simulink model "generate_elbow_motion"  (R2025a)
settings: Solver=FixedStepDiscrete  StartTime=0.0  StopTime=inf  FixedStep=0.01  RelTol=1e-3
PreLoadFcn:
  | frs = FrankaRobotSettings();
libraries: franka_simulink x1
settings Model: SimulationMode=external  ExtModeTrigDuration=10000  Creator=vasi_ko  LastModifiedBy=kvasios
settings SolverCC: ConcurrentTasks=on  AlgebraicLoopSolver=TrustRegion  AutoInsertRateTranBlk=on
settings DataIOCC: LimitDataPoints=on  SaveFormat=Array  ReturnWorkspaceOutputs=off
settings OptimizationCC: EnhancedBackFolding=on  PassReuseOutputArgsAs=Individual arguments  ZeroExternalMemoryAtStartup=off  ZeroInternalMemoryAtStartup=off  MaxStackSize=200000  OptimizeBlockOrder=speed  DifferentSizesBufferReuse=on  OptimizationCustomize=off  EfficientTunableParamExpr=on
settings DebuggingCC: SolverPrmCheckMsg=warning  ParameterTunabilityLossMsg=error  UnconnectedInputMsg=warning  UnconnectedOutputMsg=warning  UnconnectedLineMsg=warning  SFUnexpectedBacktrackingDiag=warning  SFNoUnconditionalDefaultTransitionDiag=warning  SFExecutionAtInitializationDiag=none  ArithmeticOperatorsInVariantConditions=warning
settings HardwareCC: ProdBitPerLong=64.0  ProdLargestAtomicInteger=LongLong  ProdLargestAtomicFloat=Double  ProdLongLongMode=on  ProdHWDeviceType=ARM Compatible->ARM Cortex-A (64-bit)
settings ModelReferenceCC: EnableRefExpFcnMdlSchedulingChecks=on  PropagateSignalLabelsOutOfModel=off
settings SFSimCC: SimUseLocalCustomCode=off  MATLABDynamicMemAlloc=off  CustomCodeUndefinedFunction=UseInterfaceOnly  SimTargetLang=C++  SimDLTargetLibrary=mkl-dnn
settings RTWCC: SystemTargetFile=ert.tlc  HardwareBoard=NVIDIA Jetson  TLCOptions="-aInlineSetEventsForThisBaseRateFcn=TLC_FALSE -aSuppressMultiTaskScheduler=TLC_FALSE  -aRateBasedStepFcn=0"  TemplateMakefile=ert_default_tmf  RTWVerbose=off  RTWUseLocalCustomCode=off  BuildConfiguration=Faster Runs  TargetLang=C++  GPUComputeCapability=3.5  DLArmComputeVersion=19.05  Description=Embedded Coder
settings CodeAppCC: ForceParamTrailComments=on  IgnoreCustomStorageClasses=off  OperatorAnnotations=on  SimulinkDataObjDesc=on  SFDataObjDesc=on  InsertBlockDesc=on
settings ERTTargetCC: ExtModeTransport=0.0  ExtModeMexFile=ext_comm  ExtModeIntrfLevel=Level1  InlinedParameterPlacement=Hierarchical  RootIOFormat=Structure reference  TargetLangStandard=C++14 (ISO)
settings ConfigComp: CovMetricSettings=dw  CovSaveCumulativeToWorkspaceVar=on  CovSaveSingleToWorkspaceVar=on  CovExternalEMLEnable=off  CovSFcnEnable=off

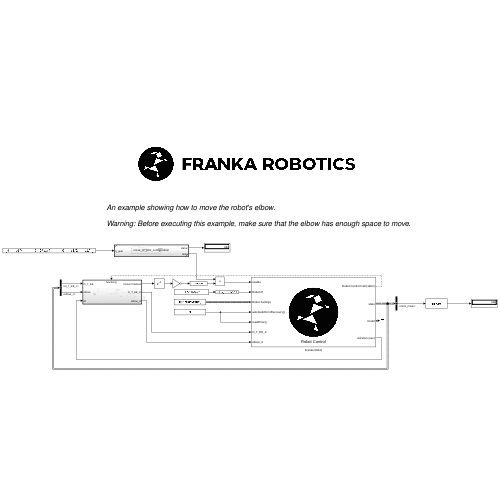
[thumbnail: Simulink's stored preview of the top-level diagram]
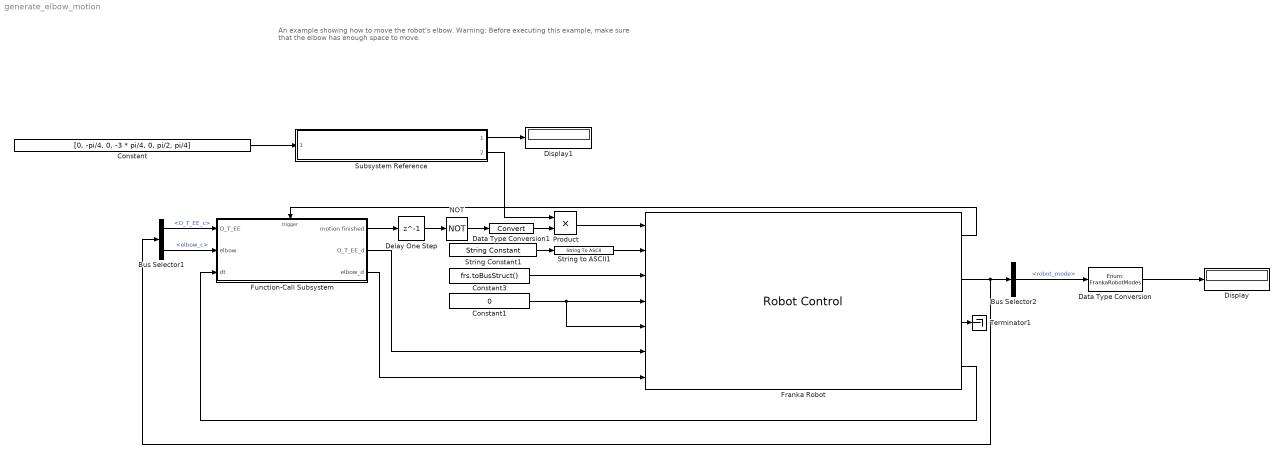
== system generate_elbow_motion ==
  note: An example showing how to move the robot's elbow.
      |
      | Warning: Before executing this example, make sure that the elbow has enough space to move.
  Bus Selector1 : BusSelector  OutputSignals=O_T_EE_c,elbow_c
  Bus Selector2 : BusSelector  OutputSignals=robot_mode
  Constant : Constant  Value=[0, -pi/4, 0, -3 * pi/4, 0, pi/2, pi/4]
  Constant1 : Constant  Value=0  OutDataTypeStr=Inherit: Inherit via back propagation
  Constant3 : Constant  Value=frs.toBusStruct()  OutDataTypeStr=Bus: FrankaRobotSettingsBus
  Data Type Conversion : DataTypeConversion  OutDataTypeStr=Enum: FrankaRobotModes  SaturateOnIntegerOverflow=off  RndMeth=Floor
  Data Type Conversion1 : DataTypeConversion  SaturateOnIntegerOverflow=off  RndMeth=Floor
  Delay One Step : Delay  DelayLength=1
  Display : Display
  Display1 : Display
  Franka Robot : franka_simulink/Robot Control  control_mode=Cartesian Pose
      settings: SourceProductName=Franka Robotics Simulink Support Package
  Function-Call Subsystem : Subsystem  TreatAsAtomicUnit=on
      settings: RTWSystemCode=Nonreusable function
  NOT : Logic  Operator=NOT  IconShape=distinctive  AllPortsSameDT=off  OutDataTypeStr=boolean
  Product : Product
  String Constant1 : StringConstant  String="\"172.16.0.2\""
  String to ASCII1 : StringToASCII  OutputVectorSize=16
  Subsystem Reference : Subsystem  TreatAsAtomicUnit=on  ReferencedSubsystem=move_to_joint_configuration
  Terminator1 : Terminator
  wires:
  Constant/1 -> Subsystem Reference/1
  Bus Selector2/1 -> Data Type Conversion/1  "<robot_mode>"
  Constant3/1 -> Franka Robot/3
  Franka Robot/4 -> Function-Call Subsystem/3(dt)
  Product/1 -> Franka Robot/1
  Function-Call Subsystem/1(motion finished) -> Delay One Step/1
  Constant1/1 -> Franka Robot/5, Franka Robot/4
  NOT/1 -> Data Type Conversion1/1
  Data Type Conversion1/1 -> Product/2
  Franka Robot/3 -> Terminator1/1
  Bus Selector1/1 -> Function-Call Subsystem/1(O_T_EE)  "<O_T_EE_c>"
  Function-Call Subsystem/2(O_T_EE_d) -> Franka Robot/6
  Subsystem Reference/2 -> Product/1
  Franka Robot/1 -> Function-Call Subsystem/Trigger
  Delay One Step/1 -> NOT/1
  Data Type Conversion/1 -> Display/1
  Franka Robot/2 -> Bus Selector1/1, Bus Selector2/1
  String Constant1/1 -> String to ASCII1/1
  Subsystem Reference/1 -> Display1/1
  String to ASCII1/1 -> Franka Robot/2
  Function-Call Subsystem/3(elbow_d) -> Franka Robot/7
  Bus Selector1/2 -> Function-Call Subsystem/2(elbow)  "<elbow_c>"

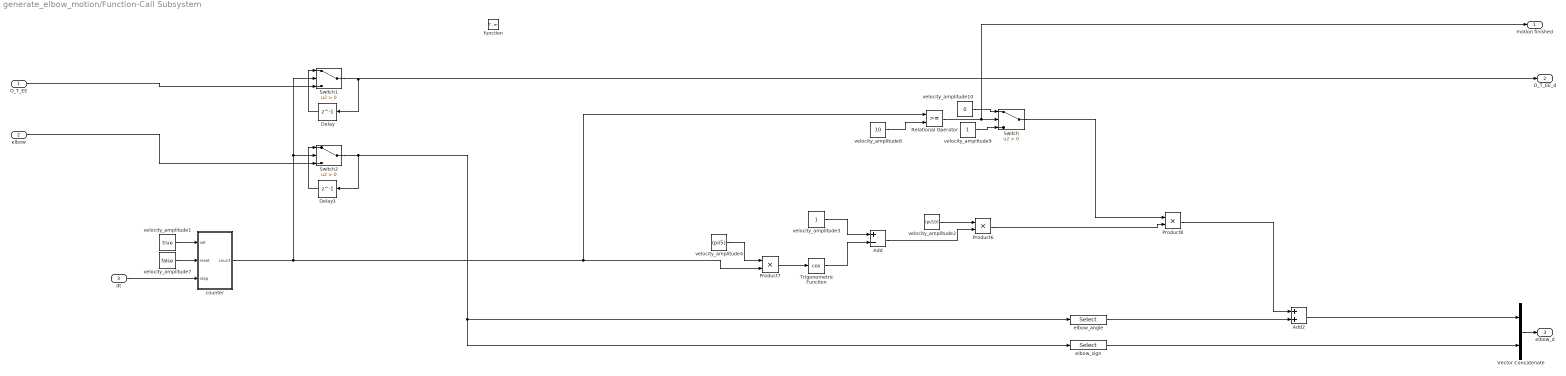
== system generate_elbow_motion/Function-Call Subsystem ==
  O_T_EE : Inport
  elbow : Inport  Port=2
  dt : Inport  Port=3
  function : TriggerPort  TriggerType=function-call  VariantControl=(inherit)
  Add : Sum  Inputs=+-
  Add2 : Sum
  Delay : Delay  DelayLength=1
  Delay1 : Delay  DelayLength=1
  Product6 : Product
  Product7 : Product
  Product8 : Product
  Relational Operator : RelationalOperator  OutDataTypeStr=boolean  InputSameDT=off
  Switch : Switch  Criteria=u2 > Threshold  SaturateOnIntegerOverflow=off  InputSameDT=off
  Switch1 : Switch  Criteria=u2 > Threshold  SaturateOnIntegerOverflow=off  InputSameDT=off
  Switch2 : Switch  Criteria=u2 > Threshold  SaturateOnIntegerOverflow=off  InputSameDT=off
  Trigonometric Function : Trigonometry  Operator=cos  NumberOfIterations=50
  Vector Concatenate : Concatenate
  counter : Subsystem
  elbow_angle : Selector  InputPortWidth=2  IndexOptions=Index vector (dialog)  Indices=1  OutputSizes=1
  elbow_sign : Selector  InputPortWidth=2  IndexOptions=Index vector (dialog)  Indices=2  OutputSizes=1
  velocity_amplitude1 : Constant  Value=true  VectorParams1D=off
  velocity_amplitude10 : Constant  Value=0  VectorParams1D=off
  velocity_amplitude2 : Constant  Value=(pi/10)  VectorParams1D=off
  velocity_amplitude3 : Constant  VectorParams1D=off
  velocity_amplitude4 : Constant  Value=(pi/5)  VectorParams1D=off
  velocity_amplitude7 : Constant  Value=false  VectorParams1D=off
  velocity_amplitude8 : Constant  Value=10  VectorParams1D=off
  velocity_amplitude9 : Constant  VectorParams1D=off
  motion finished : Outport  VectorParamsAs1DForOutWhenUnconnected=off
  O_T_EE_d : Outport  Port=2  VectorParamsAs1DForOutWhenUnconnected=off
  elbow_d : Outport  Port=3  VectorParamsAs1DForOutWhenUnconnected=off
  wires:
  elbow_angle/1 -> Add2/2
  elbow/1 -> Switch2/3
  Add/1 -> Product6/2
  velocity_amplitude7/1 -> counter/2(reset)
  counter/1(count) -> Relational Operator/1, Product7/2, Switch1/2, Switch2/2
  elbow_sign/1 -> Vector Concatenate/2
  Delay/1 -> Switch1/1
  Switch2/1 -> elbow_angle/1, elbow_sign/1, Delay1/1
  velocity_amplitude8/1 -> Relational Operator/2
  Switch1/1 -> O_T_EE_d/1, Delay/1
  velocity_amplitude4/1 -> Product7/1
  Product8/1 -> Add2/1
  velocity_amplitude9/1 -> Switch/3
  O_T_EE/1 -> Switch1/3
  Trigonometric Function/1 -> Add/2
  Switch/1 -> Product8/1
  Delay1/1 -> Switch2/1
  velocity_amplitude10/1 -> Switch/1
  Relational Operator/1 -> motion finished/1, Switch/2
  velocity_amplitude3/1 -> Add/1
  velocity_amplitude1/1 -> counter/1(set)
  Add2/1 -> Vector Concatenate/1
  Product6/1 -> Product8/2
  Product7/1 -> Trigonometric Function/1
  Vector Concatenate/1 -> elbow_d/1
  dt/1 -> counter/3(step)
  velocity_amplitude2/1 -> Product6/1

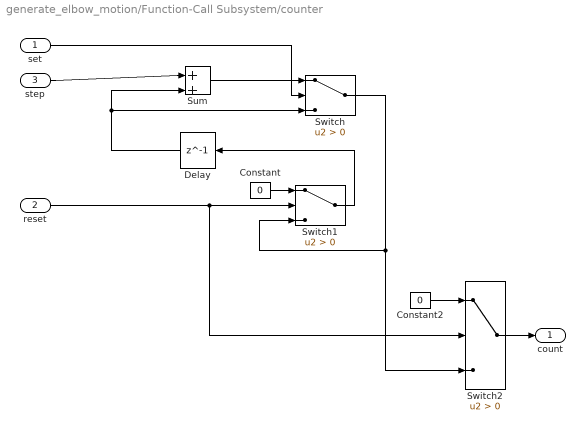
== system generate_elbow_motion/Function-Call Subsystem/counter ==
  set : Inport  OutDataTypeStr=boolean
  reset : Inport  Port=2  OutDataTypeStr=boolean
  step : Inport  Port=3  OutDataTypeStr=double
  Constant : Constant  Value=0  OutDataTypeStr=double
  Constant2 : Constant  Value=0  OutDataTypeStr=double
  Delay : Delay  DelayLength=1  InitialCondition=0
  Sum : Sum  Inputs=|++
  Switch : Switch  Criteria=u2 > Threshold  SaturateOnIntegerOverflow=off  InputSameDT=off
  Switch1 : Switch  Criteria=u2 > Threshold  OutDataTypeStr=double  SaturateOnIntegerOverflow=off  InputSameDT=off
  Switch2 : Switch  Criteria=u2 > Threshold  OutDataTypeStr=double  SaturateOnIntegerOverflow=off  InputSameDT=off
  count : Outport  OutDataTypeStr=double  VectorParamsAs1DForOutWhenUnconnected=off
  wires:
  Switch1/1 -> Delay/1
  Constant/1 -> Switch1/1
  reset/1 -> Switch2/2, Switch1/2
  Delay/1 -> Switch/3, Sum/2
  step/1 -> Sum/1
  Switch/1 -> Switch2/3, Switch1/3
  set/1 -> Switch/2
  Sum/1 -> Switch/1
  Constant2/1 -> Switch2/1
  Switch2/1 -> count/1
